simulink model "BodyCtrl_V1_1"  (R2018a)
settings: Solver=FixedStepDiscrete  StartTime=0.0  StopTime=10.0  FixedStep=sampletime  RelTol=1e-3  EnableMultiTasking=on
PreLoadFcn:
  | BodyCtrl_V1_BusInfo
libraries: simulink x2
settings Model: Creator=IAEC nishito  LastModifiedBy=E00026
settings DataIOCC: LimitDataPoints=on  SaveFormat=Array  SignalLoggingSaveFormat=ModelDataLogs  SaveOutput=off
settings OptimizationCC: DefaultParameterBehavior=Inlined  ExpressionDepthLimit=2147483647  LifeSpan=inf
settings DebuggingCC: UnderspecifiedInitializationDetection=Classic  MergeDetectMultiDrivingBlocksExec=none  SolverPrmCheckMsg=warning  FcnCallInpInsideContextMsg=warning  StateNameClashWarn=warning  SFUnexpectedBacktrackingDiag=warning  SFNoUnconditionalDefaultTransitionDiag=warning  SFExecutionAtInitializationDiag=none
settings HardwareCC: ProdBitPerPointer=32  ProdBitPerSizeT=32  ProdBitPerPtrDiffT=32  ProdLargestAtomicFloat=None  ProdIntDivRoundTo=Undefined  ProdEndianess=Unspecified  ProdWordSize=32  ProdHWDeviceType=32-bit Generic
settings ModelReferenceCC: UpdateModelReferenceTargets=IfOutOfDate  PropagateSignalLabelsOutOfModel=off
settings CodeAppCC: StateflowObjectComments=on
settings GRTTargetCC: TargetLangStandard=C89/C90 (ANSI)  GeneratePreprocessorConditionals=Disable all  CombineOutputUpdateFcns=off  GRTInterface=on
settings ConfigComp: CovMetricSettings=dw  CovHtmlReporting=on  CovSaveCumulativeToWorkspaceVar=on  CovSaveSingleToWorkspaceVar=on  CovExternalEMLEnable=off  CovSFcnEnable=off

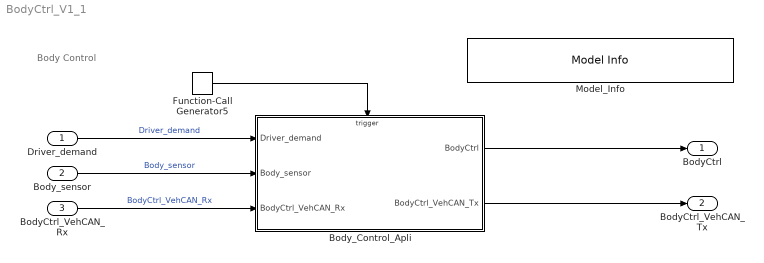
== system BodyCtrl_V1_1 ==
  note: Body Control
  Driver_demand : Inport  OutDataTypeStr=Bus: Driver_demand_Bus
      settings: AttributesFormatString=<%<OutDataTypeStr>>
  Body_sensor : Inport  Port=2  OutDataTypeStr=Bus: Body_sensor_Bus
      settings: AttributesFormatString=<%<OutDataTypeStr>>
  BodyCtrl_VehCAN_Rx : Inport  Port=3  OutDataTypeStr=Bus: BodyCtrl_VehCAN_Rx_Bus
      settings: AttributesFormatString=<%<OutDataTypeStr>>
  Body_Control_Apli : Subsystem
  Function-Call Generator5 : simulink/Ports & Subsystems/Function-Call Generator  sample_time=0.05  numberOfIterations=1
      settings: AttributesFormatString=<sample_time=%<sample_time>>
  Model_Info : simulink/Model-Wide Utilities/Model Info  Frame=on  DisplayStringWithTags=|  HorizontalTextAlignment=Left  LeftAlignmentValue=0.02
      | Version  %<ModelVersion>
      | LastModifided by %<LastModifiedBy>  Date %<LastModificationDate>
      | Description  %<Description>
  BodyCtrl : Outport  OutDataTypeStr=Bus: BodyCtrl_Bus
      settings: AttributesFormatString=<%<OutDataTypeStr>>
  BodyCtrl_VehCAN_Tx : Outport  Port=2  OutDataTypeStr=Bus: BodyCtrl_VehCAN_Tx_Bus
      settings: AttributesFormatString=<%<OutDataTypeStr>>
  wires:
  Body_Control_Apli/2(BodyCtrl_VehCAN_Tx) -> BodyCtrl_VehCAN_Tx/1
  BodyCtrl_VehCAN_Rx/1 -> Body_Control_Apli/3(BodyCtrl_VehCAN_Rx)  "BodyCtrl_VehCAN_Rx"
  Driver_demand/1 -> Body_Control_Apli/1(Driver_demand)  "Driver_demand"
  Body_Control_Apli/1(BodyCtrl) -> BodyCtrl/1
  Function-Call Generator5/1 -> Body_Control_Apli/Trigger
  Body_sensor/1 -> Body_Control_Apli/2(Body_sensor)  "Body_sensor"

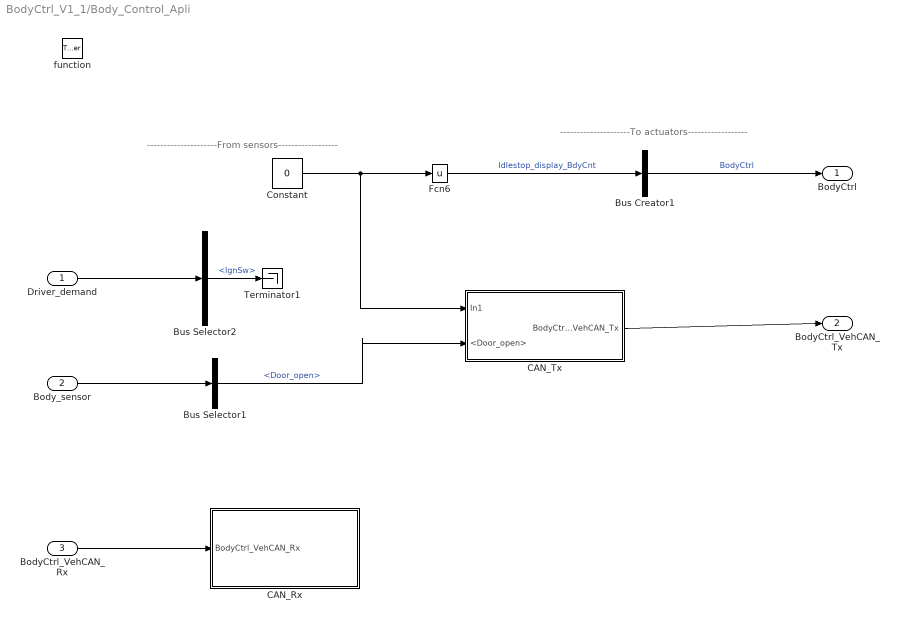
== system BodyCtrl_V1_1/Body_Control_Apli ==
  note: ---------------------From sensors------------------
  note: ---------------------To actuators------------------
  Driver_demand : Inport
  Body_sensor : Inport  Port=2
  BodyCtrl_VehCAN_Rx : Inport  Port=3
  function : TriggerPort  TriggerType=function-call  VariantControl=Variant
  Bus Creator1 : BusCreator  Inputs=1  OutDataTypeStr=Bus: BodyCtrl_Bus
      settings: AttributesFormatString=<%<OutDataTypeStr>>
  Bus Selector1 : BusSelector  OutputSignals=Door_open
  Bus Selector2 : BusSelector  OutputSignals=IgnSw
  CAN_Rx : Subsystem
  CAN_Tx : Subsystem
  Constant : Constant  Value=0
  Fcn6 : Fcn  Expr=u
  Terminator1 : Terminator
  BodyCtrl : Outport
  BodyCtrl_VehCAN_Tx : Outport  Port=2
  wires:
  Driver_demand/1 -> Bus Selector2/1
  Bus Creator1/1 -> BodyCtrl/1  "BodyCtrl"
  Fcn6/1 -> Bus Creator1/1  "Idlestop_display_BdyCnt"
  Body_sensor/1 -> Bus Selector1/1
  Constant/1 -> CAN_Tx/1(In1), Fcn6/1
  Bus Selector2/1 -> Terminator1/1  "<IgnSw>"
  Bus Selector1/1 -> CAN_Tx/2(<Door_open>)  "<Door_open>"
  CAN_Tx/1(BodyCtrl_VehCAN_Tx) -> BodyCtrl_VehCAN_Tx/1
  BodyCtrl_VehCAN_Rx/1 -> CAN_Rx/1(BodyCtrl_VehCAN_Rx)

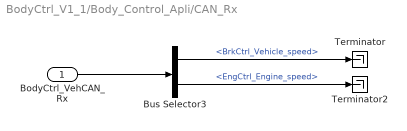
== system BodyCtrl_V1_1/Body_Control_Apli/CAN_Rx ==
  BodyCtrl_VehCAN_Rx : Inport
  Bus Selector3 : BusSelector  OutputSignals=BrkCtrl_Vehicle_speed,EngCtrl_Engine_speed
  Terminator : Terminator
  Terminator2 : Terminator
  wires:
  Bus Selector3/1 -> Terminator/1  "<BrkCtrl_Vehicle_speed>"
  BodyCtrl_VehCAN_Rx/1 -> Bus Selector3/1
  Bus Selector3/2 -> Terminator2/1  "<EngCtrl_Engine_speed>"

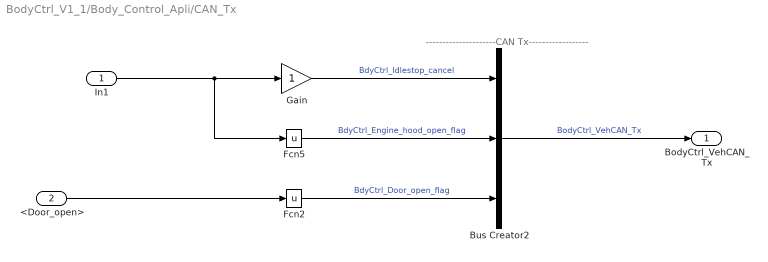
== system BodyCtrl_V1_1/Body_Control_Apli/CAN_Tx ==
  note: ---------------------CAN Tx------------------
  In1 : Inport
  <Door_open> : Inport  Port=2
  Bus Creator2 : BusCreator  Inputs=3  OutDataTypeStr=Bus: BodyCtrl_VehCAN_Tx_Bus
      settings: AttributesFormatString=<%<OutDataTypeStr>>
  Fcn2 : Fcn  Expr=u
  Fcn5 : Fcn  Expr=u
  Gain : Gain
  BodyCtrl_VehCAN_Tx : Outport
  wires:
  Fcn2/1 -> Bus Creator2/3  "BdyCtrl_Door_open_flag"
  Fcn5/1 -> Bus Creator2/2  "BdyCtrl_Engine_hood_open_flag"
  Bus Creator2/1 -> BodyCtrl_VehCAN_Tx/1  "BodyCtrl_VehCAN_Tx"
  In1/1 -> Gain/1, Fcn5/1
  <Door_open>/1 -> Fcn2/1
  Gain/1 -> Bus Creator2/1  "BdyCtrl_Idlestop_cancel"
